simulink model "e2"  (R2024b)
settings: Solver=VariableStepAuto  StartTime=0.0  StopTime=10.0  RelTol=1e-3
libraries: simulink_extras x1
settings Model: Creator=Lenovo  LastModifiedBy=Lenovo

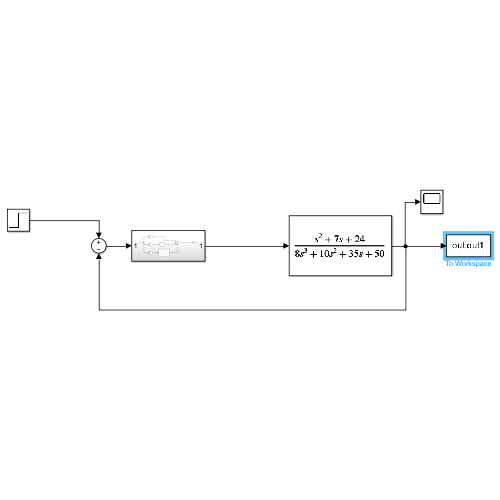
[thumbnail: Simulink's stored preview of the top-level diagram]
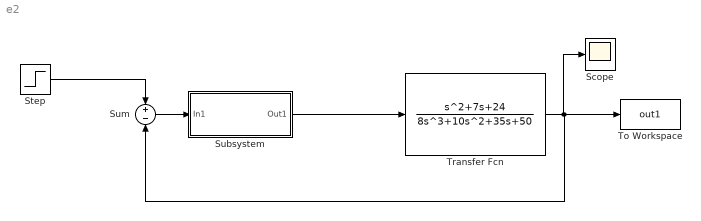
== system e2 ==
  Scope : Scope
  Step : Step  SampleTime=0
  Subsystem : Subsystem
  Sum : Sum  Inputs=+-
  To Workspace : ToWorkspace  VariableName=out1  SampleTime=-1
  Transfer Fcn : TransferFcn  Numerator=[1 7 24]  Denominator=[8 10 35 50]
  wires:
  Sum/1 -> Subsystem/1(In1)
  Subsystem/1(Out1) -> Transfer Fcn/1
  Transfer Fcn/1 -> Scope/1, Sum/2, To Workspace/1
  Step/1 -> Sum/1

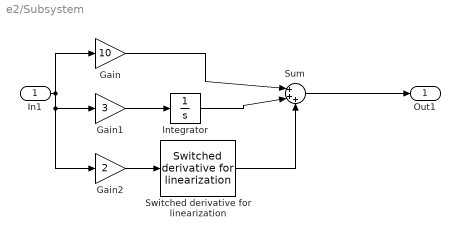
== system e2/Subsystem ==
  In1 : Inport
  Gain : Gain  Gain=10
  Gain1 : Gain  Gain=3
  Gain2 : Gain  Gain=2
  Integrator : Integrator
  Sum : Sum  Inputs=|+++
  Switched derivative for linearization : simulink_extras/Linearization/Switched derivative for linearization  switchVal=0  derivConst=100
  Out1 : Outport
  wires:
  In1/1 -> Gain2/1, Gain1/1, Gain/1
  Gain2/1 -> Switched derivative for linearization/1
  Gain1/1 -> Integrator/1
  Switched derivative for linearization/1 -> Sum/3
  Integrator/1 -> Sum/2
  Gain/1 -> Sum/1
  Sum/1 -> Out1/1
